simulink model "Demo919"  (R2018b)
settings: Solver=ode3  StartTime=0.0  StopTime=10  FixedStep=0.0005  RelTol=1e-3  EnableMultiTasking=on
values from neighbouring files (symbols this model uses):
  ADS1 = [1000 4000]    [data_new1.m]
  ADS2 = [900 4100]    [data_new1.m]
  br_opening = [0 20 40 60 80 100]    [data_new1.m]
  BRAKE = [485 1288 2091 2894 3697 4500]    [data_new1.m]
  InerWheel_Angle = [0 0.001 0.502 1.006 1.514 2.024 2.538 3.055 3.575 4.098 4.625 5.155 5.689 6.226 6.767 7.311 7.859 8.411 8.967 9.527 10.091 10.659 11.231 11.807 12.387 12.972 13.561 14.154 14.752 15.354 15.961 16.572 17.187 17.807 18.432 19.062 19.696 20.334 20.977 21.625 22.277 22.934 23.596 24.262 24.932 25.607 26.286 26.970 27.657 28.349 29.045 29.745 30.448 31.155 31.866]    [data_new1.m]
  OuterWheel_Angle = [0 0.001 0.501 1.001 1.501 2.001 2.501	3.001 3.501	4.001 4.501	5.001 5.501	6.001 6.501	7.001 7.501	8.001 8.501	9.001 9.501	10.001 10.501 11.001 11.501 12.001 12.501 13.001 13.501	14.001 14.501 15.001 15.501 16.001 16.501 17.001 17.501 18.001 18.501 19.001 19.501	20.001 20.501 21.001 21.501	22.001 22.501 23.001 23.501	24.001 24.501 25.001 25.501 26.001 26.501]    [data_new1.m]
  PUMP = [0 1000 2000 3000 4000 5000]    [data_new1.m]
  SteeringAngle_Cal = [-90 0 90]    [data_new1.m]
  SteeringAngle_Sensor = [640 1840 3041]    [data_new1.m]
  th_opening = [0 100]    [data_new1.m]
undefined symbols (not defined in the file or in its folder): D, I_AN06_5V, I_AN08_5V, I_AN09_5V, I_AN10_5V, I_HALL1, I_HALL2, I_SW01_L, I_SW10_L, I_SW11_H, I_SW12_H, I_SW13_H, I_SW14_H, I_SW15_H, I_SW16_H, I_SW17_H, I_SW18_H, I_SW19_H, I_SW20_H, O_PWM1_LS0A7, O_PWM2_LS0A7, O_SW02_LS0A4, O_SW13_HS1A, O_SW14_HS1A
libraries: ec5744lib x137, simulink x20, canmsglib x11
(part 5 of 5)

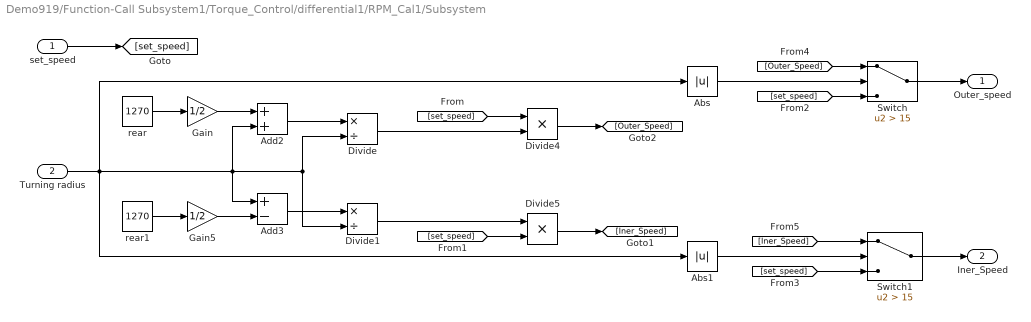
== system Demo919/Function-Call Subsystem1/Torque_Control/differential1/RPM_Cal1/Subsystem ==
  set_speed : Inport
  Turning radius : Inport  Port=2
  Abs : Abs
  Abs1 : Abs
  Add2 : Sum
  Add3 : Sum  Inputs=+-
  Divide : Product  Inputs=*/
  Divide1 : Product  Inputs=*/
  Divide4 : Product  Inputs=**
  Divide5 : Product  Inputs=**
  Gain : Gain  Gain=1/2
  Gain5 : Gain  Gain=1/2
  Switch : Switch  Criteria=u2 > Threshold  Threshold=15
  Switch1 : Switch  Criteria=u2 > Threshold  Threshold=15
  rear : Constant  Value=1270
  rear1 : Constant  Value=1270
  Outer_speed : Outport
  Iner_Speed : Outport  Port=2
  wires:
  Add2/1 -> Divide/1
  rear/1 -> Gain/1
  Turning radius/1 -> Abs1/1, Abs/1, Add2/2, Divide/2, Divide1/2, Add3/1
  Gain5/1 -> Add3/2
  Divide/1 -> Divide4/2
  Add3/1 -> Divide1/1
  rear1/1 -> Gain5/1
  Gain/1 -> Add2/1
  [set_speed] -> Divide5/2
  Divide1/1 -> Divide5/1
  [set_speed] -> Divide4/1
  Divide5/1 -> [Iner_Speed]
  Abs/1 -> Switch/2
  set_speed/1 -> [set_speed]
  [set_speed] -> Switch/3
  Switch/1 -> Outer_speed/1
  Abs1/1 -> Switch1/2
  [set_speed] -> Switch1/3
  Divide4/1 -> [Outer_Speed]
  Switch1/1 -> Iner_Speed/1
  [Outer_Speed] -> Switch/1
  [Iner_Speed] -> Switch1/1

== system Demo919/Function-Call Subsystem1/Torque_Control/differential1/RPM_Cal1/Tire_perimeter ==
  Gain1 : Gain  Gain=2
  Gain2 : Gain  Gain=pi
  tire_R : Constant  Value=0.2286
  D : Outport
  wires:
  Gain1/1 -> Gain2/1
  tire_R/1 -> Gain1/1
  Gain2/1 -> D/1

== system Demo919/Function-Call Subsystem1/Torque_Control/differential1/RPM_Cal1/Tire_perimeter1 ==
  Gain1 : Gain  Gain=2
  Gain2 : Gain  Gain=pi
  tire_R : Constant  Value=0.2286
  D : Outport
  wires:
  Gain1/1 -> Gain2/1
  tire_R/1 -> Gain1/1
  Gain2/1 -> D/1

== stateflow chart Demo919/Function-Call Subsystem1/Torque_Control/Subsystem1/AcPed_Reliable ==
  (default) -> (junction 179)
  (junction 179) -> (junction 176) [order 1] : [ Pedal_TrH < Pedal_TrL]
  (junction 179) -> (junction 177) [order 2] : {Pedal_WrongState = 0;}
  (junction 176) -> (junction 181) : {Pedal_WrongState = 1;
      | }
  (junction 181) -> (junction 177)
  (junction 177) -> (junction 184)
  data: Pedal_TrL input double; Pedal_TrH input double; Pedal_WrongState output boolean

== stateflow chart Demo919/Function-Call Subsystem1/Torque_Control/kongzhimokuai/Chart ==
  (default) -> (junction 3)
  (junction 3) -> (junction 5) [order 1] : [input<=0]
  (junction 5) -> (junction 7) : {output=eps;}
  (junction 3) -> (junction 7) [order 2] : {output=input;}
  data: input input; output output

== stateflow chart Demo919/Function-Call Subsystem1/Subsystem/WaitStart&Brake_LED ==
  note: /*检测母线电压*/
  state Main_Sf
    state HV_OFF
      en:
      Wait_Start = 0;
      RS_Rdyfg = 0;
    state HV_ON
      state WsD
      state WSE
        du:
        Wait_Start = 1;
      (default) -> WsD
      WsD -> WSE : [Key == 0 &&  Brake>=0]
    (default) -> HV_OFF
    HV_OFF -> HV_ON : [MCU1_rdy == 3&&MCU2_rdy == 3 ]
    HV_ON -> HV_OFF : [MCU1_rdy == 0&&MCU2_rdy == 0]
  note: /*待驾驶*/
  (default) -> Main_Sf
  Main_Sf -> (junction 249)
  (junction 249) -> (junction 250) [order 1] : [Brake >=5 ]
  (junction 249) -> (junction 253) [order 2] : {Break_LED = 0;
      | }
  (junction 250) -> (junction 254) : {Break_LED = 1;}
  (junction 254) -> (junction 253)
  (junction 253) -> (junction 179) : {RS_Rdyfg = 1;}
  (junction 179) -> (junction 180) [order 1] : [RS_Rdyfg == 0]
  (junction 180) -> (junction 182) : {RS = 0;}
  (junction 179) -> (junction 181) [order 2]
  (junction 182) -> (junction 181)
  (junction 181) -> (junction 121)
  (junction 121) -> (junction 138) [order 1] : [RS_Rdyfg != 0 && Wait_Start != 0]
  (junction 121) -> (junction 140) [order 2]
  (junction 138) -> (junction 139) : {WS_Sig = 1;
      | RS++;}
  (junction 139) -> (junction 140)
  (junction 140) -> (junction 141)
  (junction 141) -> (junction 147) [order 1] : [RS_Rdyfg != 0 && RS >= 300]
  (junction 141) -> (junction 149) [order 2]
  (junction 147) -> (junction 148) : {WS_Sig = 0;
      | }
  (junction 148) -> (junction 149)
  (junction 149) -> (junction 193)
  (junction 193) -> (junction 198) [order 1] : [RS >= 300]
  (junction 193) -> (junction 189) [order 2]
  (junction 198) -> (junction 199) : {RS = 300;}
  (junction 199) -> (junction 189)
  (junction 189) -> (junction 194)
  data: Brake input uint8; Wait_Start output boolean =0; Key input boolean; Break_LED output boolean; MCU1_rdy input; MCU2_rdy input; WS_Sig output boolean; RS_Rdyfg local double; RS output uint16 =0; DC_BusVolt1 input double; DC_BusVolt2 input double

== stateflow chart Demo919/Function-Call Subsystem1/Torque_Control/Subsystem1/AcPed_Reliable1 ==
  (default) -> (junction 166)
  (junction 166) -> (junction 170) [order 1] : [ Brake > 555]
  (junction 166) -> (junction 167) [order 2] : {Pedal_WrongState = 0;}
  (junction 170) -> (junction 168) : {Pedal_WrongState = 1;}
  (junction 168) -> (junction 167)
  (junction 167) -> (junction 176)
  (junction 176) -> (junction 178) [order 1] : [Brake ==0]
  (junction 176) -> (junction 180) [order 2] : {Pedal_WrongState = 0;}
  (junction 178) -> (junction 179) : {Pedal_WrongState = 1;}
  (junction 179) -> (junction 180)
  (junction 180) -> (junction 185)
  data: Pedal_WrongState output boolean; Brake input uint16

== stateflow chart Demo919/Function-Call Subsystem1/Torque_Control/Subsystem1/Ac_Arbitrate ==
  (default) -> (junction 14) : /* 油门信号仲裁 */
  (junction 14) -> (junction 15) [order 1] : [Pedal_TrL>Pedal_TrH]
  (junction 14) -> (junction 16) [order 2] : {
      | Pedal_Tr = Pedal_TrL;
      | }
  (junction 15) -> (junction 17) : {
      | Pedal_Tr = Pedal_TrH;
      | }
  (junction 17) -> (junction 16)
  (junction 16) -> (junction 18)
  data: Pedal_TrH input double; Pedal_TrL input double; Pedal_Tr output double

== stateflow chart Demo919/Function-Call Subsystem1/VCU_WrongState ==
  (default) -> (junction 29) : /*当没有报文发送时，标志位有效*/
  (junction 29) -> (junction 31)
  (junction 31) -> (junction 30) [order 1] : [VCULA == 0 || VCULB == 0]
  (junction 31) -> (junction 33) [order 2]
  (junction 30) -> (junction 32) : {CountL++;}
  (junction 32) -> (junction 33)
  (junction 33) -> (junction 39)
  (junction 39) -> (junction 59) [order 1] : [VCULA == 1 || VCULB == 1]
  (junction 39) -> (junction 57) [order 2]
  (junction 59) -> (junction 61) : {CountL = 0;}
  (junction 61) -> (junction 57)
  (junction 57) -> (junction 87)
  (junction 87) -> (junction 88) [order 1] : [VCURA == 0 || VCURB == 0]
  (junction 87) -> (junction 89) [order 2]
  (junction 88) -> (junction 83) : {CountR++;}
  (junction 83) -> (junction 89)
  (junction 89) -> (junction 82)
  (junction 82) -> (junction 90) [order 1] : [VCURA == 1 || VCURB == 1]
  (junction 82) -> (junction 86) [order 2]
  (junction 90) -> (junction 93) : {CountR = 0;}
  (junction 93) -> (junction 86)
  (junction 86) -> (junction 99)
  (junction 99) -> (junction 101) [order 1] : [CountL == 200]
  (junction 99) -> (junction 103) [order 2]
  (junction 101) -> (junction 102) : {CountL = 5;}
  (junction 102) -> (junction 103)
  (junction 103) -> (junction 112)
  (junction 112) -> (junction 116) [order 1] : [CountR == 200]
  (junction 112) -> (junction 110) [order 2]
  (junction 116) -> (junction 115) : {CountR = 5;}
  (junction 115) -> (junction 110)
  (junction 110) -> (junction 66)
  (junction 66) -> (junction 69) [order 1] : [CountL >= 5 && CountR >= 5]
  (junction 66) -> (junction 65) [order 2] : {VCU_Wo = 0;}
  (junction 69) -> (junction 70) : {VCU_Wo = 1;}
  (junction 70) -> (junction 65)
  (junction 65) -> (junction 75)
  data: VCULA input uint8; VCU_Wo output boolean; VCULB input uint8; VCURA input uint8; VCURB input uint8; CountL local uint8 =0; CountR local double =0

== stateflow chart Demo919/Function-Call Subsystem1/BMS_WrongSate ==
  (default) -> (junction 29) : /*当没有报文发送时，低边有效*/
  (junction 29) -> (junction 31)
  (junction 31) -> (junction 30) [order 1] : [BMSA == 0]
  (junction 31) -> (junction 33) [order 2]
  (junction 30) -> (junction 32) : {Count ++;}
  (junction 32) -> (junction 33)
  (junction 33) -> (junction 39)
  (junction 39) -> (junction 54) [order 1] : [BMSA == 1]
  (junction 39) -> (junction 56) [order 2]
  (junction 54) -> (junction 55) : {Count = 0;}
  (junction 55) -> (junction 56)
  (junction 56) -> (junction 73)
  (junction 73) -> (junction 75) [order 1] : [Count >= 250]
  (junction 73) -> (junction 77) [order 2]
  (junction 75) -> (junction 76) : {Count =5;}
  (junction 76) -> (junction 77)
  (junction 77) -> (junction 63)
  (junction 63) -> (junction 61) [order 1] : [Count >= 5]
  (junction 63) -> (junction 64) [order 2] : {BMS = 0;}
  (junction 61) -> (junction 66) : {BMS = 1;}
  (junction 66) -> (junction 64)
  (junction 64) -> (junction 71)
  data: BMSA input uint8; BMS output boolean; Count local uint8 =0

== stateflow chart Demo919/Function-Call Subsystem1/Chart1 ==
  state Cal
    du:
    Speed11 = (Gear_NumL/20*2*3.14*0.2286)*3.6;
    Speed12 = (Gear_NumR/20*2*3.14*0.2286)*3.6;
  (default) -> Cal
  data: Gear_NumL input double; Gear_NumR input double; Speed11 output double; Speed12 output double

== stateflow chart Demo919/Function-Call Subsystem1/Torque_Control/Subsystem1/AcPed_Reliable2 ==
  (default) -> (junction 16)
  (junction 16) -> (junction 193)
  (junction 193) -> (junction 195) [order 1] : [ Pedal_TrH - Pedal_TrL >1000]
  (junction 193) -> (junction 199) [order 2] : {Pedal_WrongState = 0;}
  (junction 195) -> (junction 197) : {Pedal_WrongState = 1;
      | }
  (junction 197) -> (junction 199)
  (junction 199) -> (junction 271)
  data: Pedal_TrL input uint16; Pedal_TrH input uint16; Pedal_WrongState output boolean

== stateflow chart Demo919/Function-Call Subsystem1/Torque_Control/kongzhimokuai/ASR_PI22/Chart2 ==
  (default) -> (junction 1)
  (junction 1) -> (junction 5) [order 1] : [a1>0.1]
  (junction 1) -> (junction 9) [order 2]
  (junction 5) -> (junction 7) : {k1=1;}
  (junction 7) -> (junction 9)
  (junction 9) -> (junction 12)
  (junction 12) -> (junction 14) [order 1] : [a1<=0.1]
  (junction 12) -> (junction 19) [order 2]
  (junction 14) -> (junction 16) : {k1=0;}
  (junction 16) -> (junction 19)
  data: a1 input; k1 output

== stateflow chart Demo919/Function-Call Subsystem1/Subsystem/Subsystem1/Chart ==
  state arithmetic
    du:
    DC_BusVolt1 = (DC_Bus_VoltH1<<8) + DC_Bus_VoltL1;
    DC_BusVolt1 = DC_BusVolt1*0.1;
  (default) -> arithmetic
  data: DC_Bus_VoltH1 input; DC_Bus_VoltL1 input; DC_BusVolt1 output double

== stateflow chart Demo919/Function-Call Subsystem1/Subsystem/Subsystem2/Chart ==
  state arithmetic
    du:
    DC_BusVolt1 = (DC_Bus_VoltH1<<8) + DC_Bus_VoltL1;
    DC_BusVolt1 = DC_BusVolt1*0.1;
  (default) -> arithmetic
  data: DC_Bus_VoltH1 input; DC_Bus_VoltL1 input; DC_BusVolt1 output double

== matlab function Demo919/Function-Call Subsystem1/Torque_Control/Kalman_Filer2/MATLAB Function ==
  data: inData input; inData_Output output; prevData input; Error input; Error_Last output
function [inData_Output,Error_Last]= fcn(inData,prevData,Error)

r = 1000;
q =70;

Error = Error + q;
kGain = Error  / ( Error  + r );                                     %//计算卡尔曼增益
inData_Output = prevData + ( kGain * ( inData - prevData ) );     %//计算本次滤波估计值
Error  = ( 1 - kGain ) * Error ;

Error_Last = Error;

== matlab function Demo919/Function-Call Subsystem1/Torque_Control/kongzhimokuai/Kalman_Filer/MATLAB Function ==
  data: inData input; inData_Output output; prevData input; Error input; Error_Last output
function [inData_Output,Error_Last]= fcn(inData,prevData,Error)

r = 1000;
q =70;

Error = Error + q;
kGain = Error  / ( Error  + r );                                     %//计算卡尔曼增益
inData_Output = prevData + ( kGain * ( inData - prevData ) );     %//计算本次滤波估计值
Error  = ( 1 - kGain ) * Error ;

Error_Last = Error;

== stateflow chart Demo919/Function-Call Subsystem1/Torque_Control/Dynamic 2 ==
  state static
    du:
    Ax_d = (AxH<<8)|AxL;
    Ay_d = (AyH<<8)|AyL;
    Az_d = (AzH<<8)|AzL;
    Ax = Ax_d/ 32768.0f * 16.0f;
    Ay = Ay_d/ 32768.0f * 16.0f;
    Az = Az_d/ 32768.0f * 16.0f;
    Yaw_d = (YawH<<8)|YawL;
    Yaw = Yaw_d/ 32768.0 * 180.0;
  (default) -> static
  data: AxL input uint8; AxH input uint8; AyL input uint8; AyH input uint8; Ax output double; Ay output double; Az output double; Ax_d output int16; Ay_d output int16; Az_d output int16; AzH input uint8; AzL input uint8; Yaw_d output int16; Yaw output double; YawH input uint8; YawL input uint8

== stateflow chart Demo919/Function-Call Subsystem1/Torque_Control/differential1/RPM_Cal1/dynamic_allocation1 ==
  note: 模式选择可以准确坐在这里，现在写的草率
  state dy_allocation2
    du:
    MAX_SPEED = 110;
  state dy_allocation1
    du:
    MAX_SPEED = 0;
  state dy_allocation3
    du:
    MAX_SPEED = 120;
  state dy_allocation4
    du:
    MAX_SPEED = 100;
  (default) -> dy_allocation1
  dy_allocation1 -> dy_allocation2 : [ MODE == 1]
  dy_allocation3 -> dy_allocation1 : [MODE == 0]
  dy_allocation2 -> dy_allocation4 : [MODE == 2]
  dy_allocation4 -> dy_allocation3 : [MODE == 3]
  data: MODE input; MAX_SPEED output uint16

== stateflow chart Demo919/Function-Call Subsystem1/Torque_Control/Chart ==
  (default) -> (junction 65) : /* 按键键码设置 */
  (junction 65) -> (junction 56) [order 1] : [Dash_Key == 2 && flg == 1]
  (junction 65) -> (junction 57) [order 2]
  (junction 56) -> (junction 51) : {Key_Num += 1;
      | flg = 0;}
  (default) -> (junction 35) [commented out] : /* 按键键码设置 */
  (junction 57) -> (junction 55) [order 1] : [Key_Num >= 4]
  (junction 57) -> (junction 69) [order 2]
  (junction 55) -> (junction 58) : {Key_Num = 0;}
  (junction 35) -> (junction 36) [commented out] : [Dash_Key == 32]
  (junction 35) -> (junction 37) [commented out]
  (junction 36) -> (junction 44) [commented out] : {Key_Num = 1;}
  (junction 69) -> (junction 71) [order 1] : [Dash_Key == 0]
  (junction 69) -> (junction 49) [order 2]
  (junction 71) -> (junction 53) : {flg = 1;}
  (junction 37) -> (junction 38) [commented out] : [Dash_Key == 16]
  (junction 37) -> (junction 39) [commented out]
  (junction 38) -> (junction 43) [commented out] : {Key_Num = 2;}
  (junction 53) -> (junction 49)
  (junction 58) -> (junction 53)
  (junction 51) -> (junction 58)
  (junction 49) -> (junction 59)
  (junction 39) -> (junction 40) [commented out] : [Dash_Key == 8]
  (junction 39) -> (junction 41) [commented out]
  (junction 40) -> (junction 42) [commented out] : {Key_Num = 3;}
  (junction 42) -> (junction 41) [commented out]
  (junction 43) -> (junction 42) [commented out]
  (junction 44) -> (junction 43) [commented out]
  (junction 41) -> (junction 45) [commented out]
  data: Dash_Key input double; Key_Num output double; flg local double

== stateflow chart Demo919/Function-Call Subsystem1/Torque_Control/Dynamic_allocation ==
  state static
    state Norm1
      en:
      Control_Command1 = 80;
      Control_Command2 = 80;
      Gear_State = 0;
      MODE = 1;
      Main_ConTactor = 1;
      du:
    state Norm
      en:
      Control_Command1 = 80;
      Control_Command2 = 80;
      Gear_State = 0;
      MODE = 0;
      Main_ConTactor = 1;
      du:
    note: 正常
    state conservation
      en:
      Control_Command1 = 80;
      Control_Command2 = 80;
      Gear_State = 0;
      MODE = 2;
      Main_ConTactor = 1;
      du:
    state Sport
      en:
      Control_Command1 = 80;
      Control_Command2 = 80;
      Gear_State = 0;
      MODE = 3;
      Main_ConTactor = 1;
      du:
    note: 节能
    note: 狂暴
    note: 可以在进入精神病模式的时候加入保险机制
    (default) -> static.Norm
    static.Norm -> static.Norm1 : [Key_Num == 1]
    static.Norm1 -> static.conservation : [Key_Num == 2]
    static.Sport -> static.Norm : [Key_Num == 0]
    static.conservation -> static.Sport : [Key_Num == 3]
  state dynamic
    state Norm
      en:
      Control_Command1 = 2;
      Control_Command2 = 2;
      Gear_State = 2;
      MODE = 0;
      Main_ConTactor = 1;
      du:
      //Mot_Speed = 2*(0*Pedal_Tr+10000);
      //Mot_Torq = 0*Pedal_Tr;
    state Norm1
      en:
      Control_Command1 = 2;
      Control_Command2 = 2;
      Gear_State = 2;
      MODE = 1;
      Main_ConTactor = 1;
      du:
      //Mot_Speed = 2*(43*Pedal_Tr+10000);
      //Mot_Torq = 7.5*Pedal_Tr;
    note: 正常
    state Sport
      en:
      Control_Command1 = 2;
      Control_Command2 = 2;
      Gear_State = 2;
      MODE = 3;
      Main_ConTactor = 1;
      du:
      //Mot_Speed = 2*(50*Pedal_Tr+10000);
      //Mot_Torq = 8*Pedal_Tr;
    state conservation
      en:
      Control_Command1 = 2;
      Control_Command2 = 2;
      Gear_State = 2;
      MODE = 2;
      Main_ConTactor = 1;
      du:
      //Mot_Speed = 2*(30*Pedal_Tr+10000);
      //Mot_Torq = 5*Pedal_Tr;
    note: 狂暴
    note: 节能
    (default) -> dynamic.Norm
    dynamic.Norm -> dynamic.Norm1 [order 1] : [Key_Num == 1]
    dynamic.Norm -> dynamic.conservation [order 2] : [Key_Num == 2]
    dynamic.Sport -> dynamic.Norm : [Key_Num == 0  ]
    dynamic.Norm -> dynamic.Sport [order 3] : [Key_Num == 3]
    dynamic.Norm1 -> dynamic.conservation : [Key_Num == 2]
    dynamic.conservation -> dynamic.Sport : [Key_Num == 3]
  state dynamic2
    state Norm
      en:
      Control_Command1 = 82;
      Control_Command2 = 82;
      Gear_State = 2;
      MODE = 0;
      Main_ConTactor = 1;
      du:
      //Mot_Speed = 2*(0*Pedal_Tr+10000);
      //Mot_Torq = 0*Pedal_Tr;
    state Norm1
      en:
      Control_Command1 = 82;
      Control_Command2 = 82;
      Gear_State = 2;
      MODE = 1;
      Main_ConTactor = 1;
      du:
      //Mot_Speed = 2*(43*Pedal_Tr+10000);
      //Mot_Torq = 7.5*Pedal_Tr;
    note: 正常
    state Sport
      en:
      Control_Command1 = 82;
      Control_Command2 = 82;
      Gear_State = 2;
      MODE = 3;
      Main_ConTactor = 1;
      du:
      //Mot_Speed = 2*(50*Pedal_Tr+10000);
      //Mot_Torq = 8*Pedal_Tr;
    state conservation
      en:
      Control_Command1 = 82;
      Control_Command2 = 82;
      Gear_State = 2;
      MODE = 2;
      Main_ConTactor = 1;
      du:
      //Mot_Speed = 2*(30*Pedal_Tr+10000);
      //Mot_Torq = 5*Pedal_Tr;
    note: 狂暴
    note: 节能
    (default) -> dynamic2.Norm
    dynamic2.Norm -> dynamic2.Norm1 [order 1] : [Key_Num == 1]
    dynamic2.Norm -> dynamic2.conservation [order 2] : [Key_Num == 2]
    dynamic2.Sport -> dynamic2.Norm : [Key_Num == 0  ]
    dynamic2.Norm -> dynamic2.Sport [order 3] : [Key_Num == 3]
    dynamic2.Norm1 -> dynamic2.conservation : [Key_Num == 2]
    dynamic2.conservation -> dynamic2.Sport : [Key_Num == 3]
  state dynamic1 [commented out]
    du:
    Control_Command1 = 82;
    Control_Command2 = 82;
    Gear_State = 2;
    Main_ConTactor = 1;
  (default) -> static
  dynamic -> static [order 2] : [Wait_Start == 0]
  static -> dynamic : [Wait_Start == 1]
  dynamic2 -> dynamic : [Pedal_WS == 0 | PEDALTR != 0 ]
  dynamic -> dynamic2 [order 1] : [Pedal_WS == 1  | PEDALTR == 0 ]
  data: Key_Num input double; PEDALTR input; Pedal_WS input; Control_Command1 output uint8; Control_Command2 output uint8; Wait_Start input boolean; MODE output uint8; Gear_State output double; Main_ConTactor output boolean

== stateflow chart Demo919/Function-Call Subsystem1/Torque_Control/kongzhimokuai/ASR_PI21/Chart1 ==
  (default) -> (junction 1)
  (junction 1) -> (junction 5) [order 1] : [a1>0.1]
  (junction 1) -> (junction 9) [order 2]
  (junction 5) -> (junction 7) : {k1=1;}
  (junction 7) -> (junction 9)
  (junction 9) -> (junction 12)
  (junction 12) -> (junction 14) [order 1] : [a1<=0.1]
  (junction 12) -> (junction 19) [order 2]
  (junction 14) -> (junction 16) : {k1=0;}
  (junction 16) -> (junction 19)
  data: a1 input; k1 output

== stateflow chart Demo919/Function-Call Subsystem1/Torque_Control/kongzhimokuai/Chart3 ==
  (default) -> (junction 3)
  (junction 3) -> (junction 5) [order 1] : [input==0]
  (junction 5) -> (junction 7) : {output=(input+(1/eps));}
  (junction 3) -> (junction 7) [order 2] : {output=input;}
  data: input input; output output

== stateflow chart Demo919/Function-Call Subsystem1/Torque_Control/kongzhimokuai/Chart1 ==
  (default) -> (junction 3)
  (junction 3) -> (junction 5) [order 1] : [input==0]
  (junction 5) -> (junction 7) : {output=(input+eps);}
  (junction 3) -> (junction 7) [order 2] : {output=input;}
  data: input input; output output

== stateflow chart Demo919/Function-Call Subsystem1/Torque_Control/kongzhimokuai/Chart2 ==
  (default) -> (junction 3)
  (junction 3) -> (junction 5) [order 1] : [input==0]
  (junction 5) -> (junction 7) : {output=(input+eps);}
  (junction 3) -> (junction 7) [order 2] : {output=input;}
  data: input input; output output

== stateflow chart Demo919/Function-Call Subsystem1/Torque_Control/differential1/dynamic_allocation ==
  state dy_allocation1
    du:
    LMot_Speed = 2*(InerMotor_RPM+10000);
    RMot_Speed = 2*(OuterMotor_RPM+10000);
  state dy_allocation2
    du:
    LMot_Speed = 2*(OuterMotor_RPM+10000);
    RMot_Speed = 2*(InerMotor_RPM+10000);
  (default) -> dy_allocation1
  dy_allocation1 -> dy_allocation2 : [LR_Flg == 1]
  dy_allocation2 -> dy_allocation1 : [LR_Flg == 0]
  data: LR_Flg input; OuterMotor_RPM input uint16; InerMotor_RPM input uint16; LMot_Speed output uint16; RMot_Speed output uint16

== stateflow chart Demo919/Function-Call Subsystem1/Torque_Control/kongzhimokuai/ASR_PI21/Chart4 ==
  (default) -> (junction 3)
  (junction 3) -> (junction 5) [order 1] : [input==0]
  (junction 5) -> (junction 7) : {output=(input+(1/eps));}
  (junction 3) -> (junction 7) [order 2] : {output=input;}
  data: input input; output output

== stateflow chart Demo919/Function-Call Subsystem1/Torque_Control/kongzhimokuai/akerman1/Chart ==
  (default) -> (junction 3)
  (junction 3) -> (junction 20) [order 3] : [-10<x<10]
  (junction 3) -> (junction 5) [order 1] : [x<=(-10)]
  (junction 20) -> (junction 10) : {y=0;}
  (junction 5) -> (junction 10) : {y=(-1);}
  (junction 3) -> (junction 7) [order 2] : [x>=10]
  (junction 7) -> (junction 10) : {y=1;}
  (junction 10) -> (junction 25)
  data: x input; y output

== matlab function Demo919/Function-Call Subsystem1/Torque_Control/kongzhimokuai/Kalman_Filer1/MATLAB Function ==
  data: inData input; inData_Output output; prevData input; Error input; Error_Last output
function [inData_Output,Error_Last]= fcn(inData,prevData,Error)

r = 1000;
q =70;

Error = Error + q;
kGain = Error  / ( Error  + r );                                     %//计算卡尔曼增益
inData_Output = prevData + ( kGain * ( inData - prevData ) );     %//计算本次滤波估计值
Error  = ( 1 - kGain ) * Error ;

Error_Last = Error;

== stateflow chart Demo919/Function-Call Subsystem1/Torque_Control/Subsystem1/AcPed_Reliable3 ==
  (default) -> (junction 16)
  (junction 16) -> (junction 193)
  (junction 193) -> (junction 195) [order 1] : [ Pedal_TrH < 100 || Pedal_TrL  < 100]
  (junction 193) -> (junction 199) [order 2] : {Pedal_WrongState = 0;}
  (junction 195) -> (junction 197) : {Pedal_WrongState = 1;
      | }
  (junction 197) -> (junction 199)
  (junction 199) -> (junction 271)
  data: Pedal_TrL input uint16; Pedal_TrH input uint16; Pedal_WrongState output boolean

== stateflow chart Demo919/Function-Call Subsystem1/Torque_Control/kongzhimokuai/ASR_PI22/Chart4 ==
  (default) -> (junction 3)
  (junction 3) -> (junction 5) [order 1] : [input==0]
  (junction 5) -> (junction 7) : {output=(input+(1/eps));}
  (junction 3) -> (junction 7) [order 2] : {output=input;}
  data: input input; output output

== matlab function Demo919/Function-Call Subsystem1/Torque_Control/Kalman_Filer3/MATLAB Function ==
  data: inData input; inData_Output output; prevData input; Error input; Error_Last output
function [inData_Output,Error_Last]= fcn(inData,prevData,Error)

r = 1000;
q =70;

Error = Error + q;
kGain = Error  / ( Error  + r );                                     %//计算卡尔曼增益
inData_Output = prevData + ( kGain * ( inData - prevData ) );     %//计算本次滤波估计值
Error  = ( 1 - kGain ) * Error ;

Error_Last = Error;

== matlab function Demo919/Function-Call Subsystem1/Torque_Control/Kalman_Filer4/MATLAB Function ==
  data: inData input; inData_Output output; prevData input; Error input; Error_Last output
function [inData_Output,Error_Last]= fcn(inData,prevData,Error)

r = 1000;
q =70;

Error = Error + q;
kGain = Error  / ( Error  + r );                                     %//计算卡尔曼增益
inData_Output = prevData + ( kGain * ( inData - prevData ) );     %//计算本次滤波估计值
Error  = ( 1 - kGain ) * Error ;

Error_Last = Error;
